simulink model "MPPIController"  (R2024b)
settings: Solver=FixedStepDiscrete  StartTime=0.0  StopTime=Inf  RelTol=1e-3
undefined symbols (not defined in the file or in its folder): fixedControllerParams, maxLocalPathLen, maxRefPathLen
settings Model: Creator=apattass  LastModifiedBy=apattass

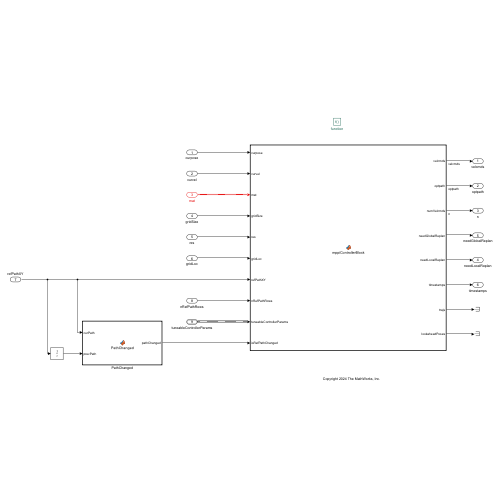
[thumbnail: Simulink's stored preview of the top-level diagram]
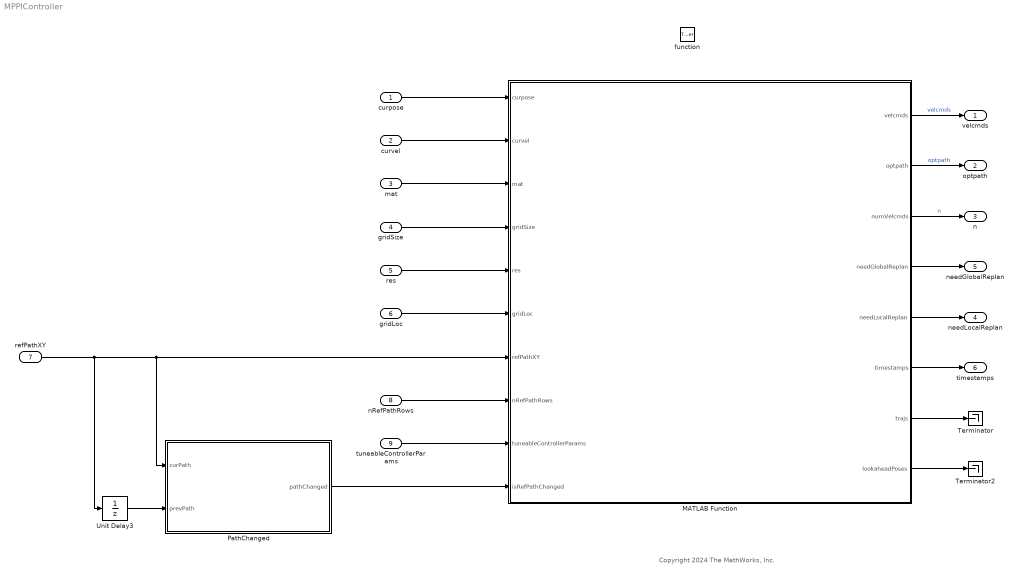
== system MPPIController ==
  note: Copyright 2024 The MathWorks, Inc.
  curpose : Inport  OutDataTypeStr=double  PortDimensions=[1 3]
  curvel : Inport  Port=2  OutDataTypeStr=double  PortDimensions=[1 2]
  mat : Inport  Port=3  OutDataTypeStr=boolean  PortDimensions=[1201 1201]  Interpolate=off
      settings: VarSizeSig=Yes
  gridSize : Inport  Port=4  PortDimensions=[1 2]
  res : Inport  Port=5  OutDataTypeStr=double  PortDimensions=1
  gridLoc : Inport  Port=6  OutDataTypeStr=double  PortDimensions=[1 2]
  refPathXY : Inport  Port=7  OutDataTypeStr=double  PortDimensions=[maxRefPathLen 3]
  nRefPathRows : Inport  Port=8  OutDataTypeStr=double  PortDimensions=1
  tuneableControllerParams : Inport  Port=9  OutDataTypeStr=Bus: controller_bus  BusOutputAsStruct=on
  function : TriggerPort  TriggerType=function-call  FunctionName=planLocalMPPI  VariantControl=(inherit)
  MATLAB Function : MATLAB Function  TreatAsAtomicUnit=on  mask{length=fixedControllerParams.Length, width=fixedControllerParams.Width, maxOutputLength=maxLocalPathLen, visualizePath=on}
      mask prompts: length "Length of vehicle (in meters)"; width "Width of vehicle (in meters)"; maxOutputLength "Maximum States In Output"; visualizePath "Visualize LocalPath?"
  PathChanged : MATLAB Function  TreatAsAtomicUnit=on
  Terminator : Terminator
  Terminator2 : Terminator
  Unit Delay3 : UnitDelay  SampleTime=-1  HasFrameUpgradeWarning=on
  velcmds : Outport  OutDataTypeStr=double  PortDimensions=[maxLocalPathLen 2]
  optpath : Outport  Port=2  OutDataTypeStr=double  PortDimensions=[maxLocalPathLen 3]
  n : Outport  Port=3  OutDataTypeStr=double  PortDimensions=1
  needLocalReplan : Outport  Port=4  OutDataTypeStr=double  PortDimensions=1
  needGlobalReplan : Outport  Port=5  OutDataTypeStr=double  PortDimensions=1
  timestamps : Outport  Port=6  PortDimensions=[maxLocalPathLen 1]
  wires:
  refPathXY/1 -> PathChanged/1(curPath), MATLAB Function/7(refPathXY), Unit Delay3/1
  gridSize/1 -> MATLAB Function/4(gridSize)
  Unit Delay3/1 -> PathChanged/2(prevPath)
  tuneableControllerParams/1 -> MATLAB Function/9(tuneableControllerParams)
  mat/1 -> MATLAB Function/3(mat)
  res/1 -> MATLAB Function/5(res)
  gridLoc/1 -> MATLAB Function/6(gridLoc)
  nRefPathRows/1 -> MATLAB Function/8(nRefPathRows)
  curpose/1 -> MATLAB Function/1(curpose)
  curvel/1 -> MATLAB Function/2(curvel)
  PathChanged/1(pathChanged) -> MATLAB Function/10(isRefPathChanged)
  MATLAB Function/2(optpath) -> optpath/1  "optpath"
  MATLAB Function/1(velcmds) -> velcmds/1  "velcmds"
  MATLAB Function/3(numVelcmds) -> n/1  "n"
  MATLAB Function/4(needGlobalReplan) -> needGlobalReplan/1
  MATLAB Function/6(timestamps) -> timestamps/1
  MATLAB Function/5(needLocalReplan) -> needLocalReplan/1
  MATLAB Function/7(trajs) -> Terminator/1
  MATLAB Function/8(lookaheadPoses) -> Terminator2/1

== matlab function MPPIController/PathChanged ==
  data: curPath input; prevPath input; pathChanged output
function pathChanged = PathChanged(curPath, prevPath)
%PathChanged Return true if new path has been provided else return false
    
pathChanged = false;
if ~isequal(curPath,prevPath)
    pathChanged = true;
end
end

== matlab function MPPIController/MATLAB Function ==
  data: curpose input; curvel input; mat input; gridSize input; res input; velcmds output; gridLoc input; refPathXY input size=[maxRefPathLen 3]; nRefPathRows input; tuneableControllerParams input Bus:controller_bus; isRefPathChanged input; optpath output; length parameter; width parameter; numVelcmds output size=[1 1]; maxOutputLength parameter; needGlobalReplan output; needLocalReplan output; timestamps output; trajs output; lookaheadPoses output
function [velcmds,optpath,numVelcmds,needGlobalReplan,needLocalReplan, timestamps, trajs,lookaheadPoses] = mppiControllerBlock(curpose, curvel, mat, gridSize, res, ...
    gridLoc, refPathXY, nRefPathRows, tuneableControllerParams, isRefPathChanged, ...
    length, width, maxOutputLength)
    
    velcmds = nan(maxOutputLength,2);
    optpath = nan(maxOutputLength,3);
    timestamps = nan(maxOutputLength,1);
    trajs = nan(200,3,500);
    lookaheadPoses = nan(5000,3);

    numVelcmds = 0;
    needGlobalReplan = 0;
    needLocalReplan = 0;
    if nRefPathRows ~= 0 
        egoMat = mat(1:gridSize(1),1:gridSize(2));

        [velcmds_,optpath_,sampleTime,needGlobalReplan,needLocalReplan,trajs_,numTraj_,lookaheadPoses_] = MPPIControllerFcn(egoMat, res, gridLoc, ...
            refPathXY(1:nRefPathRows,:), isRefPathChanged, curpose, curvel, tuneableControllerParams, ...
            length, width);       

        numVelcmds = size(velcmds_,1);
        velcmds(1:numVelcmds,:)      = velcmds_;
        optpath(1:numVelcmds,:)      = optpath_;
        timestamps(1:numVelcmds,1)   = 0:sampleTime:(numVelcmds-1)*sampleTime;
        trajs(1:numVelcmds,1:3,1:numTraj_) = trajs_;
        numLADPoses = size(lookaheadPoses_,1);
        lookaheadPoses(1:numLADPoses,:) = lookaheadPoses_;
    end
end
